simulink model "ABS_Regen_SLC_Test"  (R2023a)
settings: Solver=ode45  StartTime=0  StopTime=15  FixedStep=0.002  RelTol=1e-3  AbsTol=1e-6
libraries: Solver_SF x1, cstblocks x1
settings Model: ExtModeTrigMode=oneshot  VariantFading=off  Creator=ywata  LastModifiedBy=cheho
settings SolverCC: AutoScaleAbsTol=off  AlgebraicLoopSolver=TrustRegion
settings DataIOCC: SaveFormat=Array  SignalLoggingSaveFormat=ModelDataLogs  ReturnWorkspaceOutputs=off  SignalLoggingName=sigsOut
settings OptimizationCC: BlockReduction=off  BooleanDataType=off  ExpressionDepthLimit=2147483647  LifeSpan=inf
settings DebuggingCC: SaveWithParameterizedLinksMsg=none  UnderspecifiedInitializationDetection=Classic  MergeDetectMultiDrivingBlocksExec=none  SignalResolutionControl=TryResolveAllWithWarning  MultiTaskDSMMsg=warning  MultiTaskCondExecSysMsg=none  FcnCallInpInsideContextMsg=warning  UnconnectedInputMsg=warning  UnconnectedOutputMsg=warning  UnconnectedLineMsg=warning  StateNameClashWarn=warning  SFUnexpectedBacktrackingDiag=warning  SFNoUnconditionalDefaultTransitionDiag=warning  SFExecutionAtInitializationDiag=none  ArithmeticOperatorsInVariantConditions=warning
settings HardwareCC: ProdBitPerPointer=32  ProdBitPerSizeT=32  ProdBitPerPtrDiffT=32  ProdLargestAtomicFloat=None  ProdIntDivRoundTo=Undefined  ProdEndianess=Unspecified  ProdWordSize=32  ProdHWDeviceType=32-bit Generic  TargetUnknown=on
settings ModelReferenceCC: PropagateSignalLabelsOutOfModel=off
settings SFSimCC: SimUseLocalCustomCode=off  CustomCodeUndefinedFunction=UseInterfaceOnly
settings RTWCC: TemplateMakefile=grt_vc.tmf  RTWUseLocalCustomCode=off
settings CodeAppCC: StateflowObjectComments=on
settings GRTTargetCC: TargetFcnLib=ansi_tfl_tmw.mat  TargetLangStandard=C89/C90 (ANSI)  CombineOutputUpdateFcns=off  GRTInterface=on
settings ConfigComp: CovMetricSettings=dw  CovSaveCumulativeToWorkspaceVar=on  CovSaveSingleToWorkspaceVar=on  CovExternalEMLEnable=off

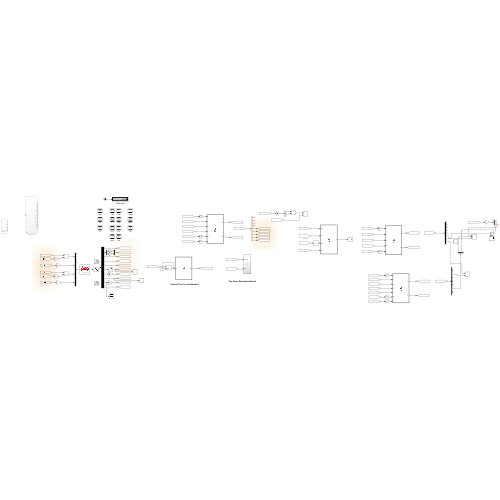
[thumbnail: Simulink's stored preview of the top-level diagram]
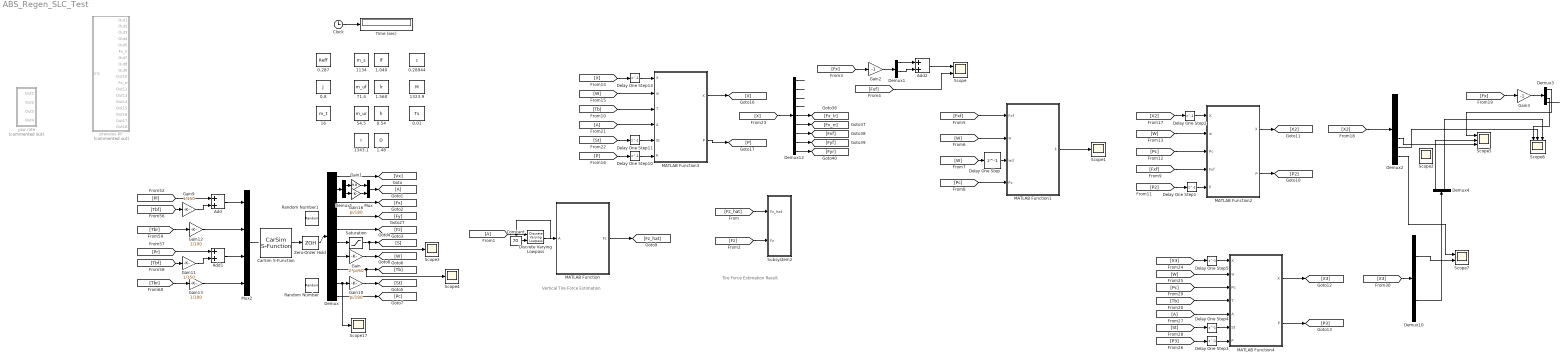
== system ABS_Regen_SLC_Test ==
  note: Vertical Tire Force Estimation
  note: Tire Force Estimation Result
  0.01 : DataStoreMemory  DataStoreName=Ts  WriteAfterWriteMsg=warning  InitialValue=0.01  ShowAdditionalParam=off  OutDataTypeStr=double
  0.287 : DataStoreMemory  DataStoreName=Reff  WriteAfterWriteMsg=warning  InitialValue=0.287  ShowAdditionalParam=off  OutDataTypeStr=double
  0.28944 : DataStoreMemory  DataStoreName=c  WriteAfterWriteMsg=warning  InitialValue=0.29844  ShowAdditionalParam=off  OutDataTypeStr=double
  0.54 : DataStoreMemory  DataStoreName=h  WriteAfterWriteMsg=warning  InitialValue=0.54  ShowAdditionalParam=off  OutDataTypeStr=double
  0.8 : DataStoreMemory  DataStoreName=J  WriteAfterWriteMsg=warning  InitialValue=0.8  ShowAdditionalParam=off  OutDataTypeStr=double
  1.040 : DataStoreMemory  DataStoreName=lf  WriteAfterWriteMsg=warning  InitialValue=1.040  ShowAdditionalParam=off  OutDataTypeStr=double
  1.48 : DataStoreMemory  DataStoreName=D  WriteAfterWriteMsg=warning  InitialValue=1.48  ShowAdditionalParam=off  OutDataTypeStr=double
  1.560 : DataStoreMemory  DataStoreName=lr  WriteAfterWriteMsg=warning  InitialValue=1.560  ShowAdditionalParam=off  OutDataTypeStr=double
  1134 : DataStoreMemory  DataStoreName=m_s  WriteAfterWriteMsg=warning  InitialValue=1134  ShowAdditionalParam=off  OutDataTypeStr=double
  1323.9 : DataStoreMemory  DataStoreName=M  WriteAfterWriteMsg=warning  InitialValue=1323.9  ShowAdditionalParam=off  OutDataTypeStr=double
  1343.1 : DataStoreMemory  DataStoreName=I  WriteAfterWriteMsg=warning  InitialValue=1343.1  ShowAdditionalParam=off  OutDataTypeStr=double
  16 : DataStoreMemory  DataStoreName=m_t  WriteAfterWriteMsg=warning  InitialValue=16  ShowAdditionalParam=off  OutDataTypeStr=double
  54.5 : DataStoreMemory  DataStoreName=m_ur  WriteAfterWriteMsg=warning  InitialValue=54.5  ShowAdditionalParam=off  OutDataTypeStr=double
  71.4 : DataStoreMemory  DataStoreName=m_uf  WriteAfterWriteMsg=warning  InitialValue=71.4  ShowAdditionalParam=off  OutDataTypeStr=double
  Add : Sum
  Add1 : Sum
  Add2 : Sum
  CarSim S-Function : Solver_SF/CarSim S-Function  Priority=1  SIMFILE=simfile.sim  Run_RTs=off  vs_state_ind=Run  StopMode_ind=Vehicle Model
  Clock : Clock
  Constant : Constant  Value=70  SampleTime=0.01
  Delay One Step : Delay  DelayLength=1  InitialCondition=[67.665 67.665 67.665 67.665]'
  Delay One Step1 : Delay  DelayLength=1  InitialCondition=diag([67.655 67.655 0 0 0 0 0])
  Delay One Step10 : Delay  DelayLength=1  InitialCondition=diag([67.655 67.655 0 0 0 0 0 0 0])
  Delay One Step11 : Delay  DelayLength=1  InitialCondition=[0 0]'
  Delay One Step14 : Delay  DelayLength=1  InitialCondition=[67.655 67.655 0 0 0 0 0 0 0]'
  Delay One Step2 : Delay  DelayLength=1  InitialCondition=[67.655 67.655 0 0 0 0 0]'
  Delay One Step3 : Delay  DelayLength=1  InitialCondition=diag([67.655 67.655 67.655 67.655 250 0 0 0 0 0 0 0 0 0 0 0])
  Delay One Step4 : Delay  DelayLength=1  InitialCondition=[0 0]'
  Delay One Step5 : Delay  DelayLength=1  InitialCondition=[67.655 67.655 67.655 67.655 100 0 0 0 0 0 0 0 0 0 0 0]'
  Demux : Demux  Outputs=[1 3 4 4 4 4 4 4 2 2]
  Demux1 : Demux
  Demux10 : Demux  Outputs=[4 1 2 1 2 4 2]
  Demux12 : Demux  Outputs=9
  Demux2 : Demux  Outputs=7
  Demux3 : Demux
  Demux4 : Demux
  Demux5 : Demux  Outputs=[2 1]
  Discrete Varying Lowpass : cstblocks/Linear Parameter Varying/Discrete Varying Lowpass  N=1  w0=0  Ts=0.01
  From1 : From
  From21 : From
  From27 : From
  Gain : Gain  Gain=2*pi/60
  Gain1 : Gain  Gain=9.8
  Gain10 : Gain  Gain=pi/180
  Gain11 : Gain  Gain=1/150
  Gain12 : Gain  Gain=1/100
  Gain13 : Gain  Gain=1/100
  Gain16 : Gain  Gain=pi/180
  Gain2 : Gain  Gain=-1
  Gain3 : Gain  Gain=-1
  Gain9 : Gain  Gain=1/150
  Goto1 : Goto
  MATLAB Function : MATLAB Function  TreatAsAtomicUnit=on
  MATLAB Function1 : MATLAB Function  TreatAsAtomicUnit=on
  MATLAB Function2 : MATLAB Function  TreatAsAtomicUnit=on
  MATLAB Function3 : MATLAB Function  TreatAsAtomicUnit=on
  MATLAB Function4 : MATLAB Function  TreatAsAtomicUnit=on
  Mux : Mux  Inputs=2
  Mux2 : Mux
  Random Number : RandomNumber  Variance=0.01^2  SampleTime=0.01
  Random Number1 : RandomNumber  Variance=0.01  SampleTime=0.01
  Saturation : Saturate  UpperLimit=1  LowerLimit=-1
  Scope : Scope  NumInputPorts=2
  Scope{1..4,17} (5 alike) : Scope
  Scope5 : Scope  NumInputPorts=3
  Scope6 : Scope  NumInputPorts=3
  Scope7 : Scope  NumInputPorts=2
  Subsystem2 : Subsystem
  Time (sec) : Display
      settings: Format=bank  Decimation=100
  Zero-Order Hold : ZeroOrderHold  SampleTime=0.01
  previous KF : Subsystem  Commented=on
  yaw rate : Subsystem  Commented=on
  wires:
  CarSim S-Function/1 -> Zero-Order Hold/1
  Clock/1 -> Time (sec)/1
  Demux/1 -> [Vx]
  Demux/3 -> [Fx]
  Zero-Order Hold/1 -> Demux/1
  Saturation/1 -> Scope3/1, [S]
  Gain/1 -> [W]
  Demux/2 -> Demux5/1
  Demux5/1 -> Gain1/1
  Mux/1 -> Goto1/1
  Demux5/2 -> Gain16/1
  Gain1/1 -> Mux/1
  Demux/10 -> [Pc]
  Demux/9 -> Scope17/1, Gain10/1
  Demux/8 -> Scope4/1, [Tb]
  Demux/7 -> Gain/1
  Demux/6 -> Saturation/1
  Demux/5 -> [Fz]
  Demux/4 -> [Fy]
  Gain16/1 -> Mux/2
  Gain10/1 -> [St]
  From1/1 -> MATLAB Function/1(A), Discrete Varying Lowpass/1
  MATLAB Function/1(Fz) -> [Fz_hat]
  [Fz_hat] -> Subsystem2/1(Fz_hat)
  [Fz] -> Subsystem2/2(Fz)
  Constant/1 -> Discrete Varying Lowpass/2
  Discrete Varying Lowpass/1 -> ?
  Add/1 -> Mux2/1
  [Pl] -> Add/1
  [Tbf] -> Gain9/1
  Gain9/1 -> Add/2
  [Tbf] -> Gain11/1
  Add1/1 -> Mux2/3
  [Pr] -> Add1/1
  Gain11/1 -> Add1/2
  [Tbr] -> Gain12/1
  Gain12/1 -> Mux2/2
  Gain13/1 -> Mux2/4
  [Tbr] -> Gain13/1
  Mux2/1 -> ?
  [P] -> Delay One Step10/1
  Demux12/3 -> ?
  [X] -> Demux12/1
  Demux12/1 -> ?
  Demux12/2 -> ?
  Delay One Step14/1 -> MATLAB Function3/1("X ")
  Demux12/4 -> ?
  Demux12/8 -> [Fyf]
  Demux12/9 -> [Fyr]
  Delay One Step10/1 -> MATLAB Function3/6("P ")
  Demux12/6 -> [Fx_rr]
  [Tb] -> MATLAB Function3/3(T)
  MATLAB Function3/2(P) -> [P]
  Delay One Step11/1 -> MATLAB Function3/5(St)
  [W] -> MATLAB Function3/2(w)
  MATLAB Function3/1(X) -> [X]
  [X] -> Delay One Step14/1
  Demux12/5 -> [Fx_lr]
  From21/1 -> MATLAB Function3/4(A)
  Demux12/7 -> [Fxf]
  [St] -> Delay One Step11/1
  [Fx] -> Gain2/1
  Demux1/1 -> Add2/1
  Demux1/3 -> Add2/2
  Add2/1 -> Scope/1
  Gain2/1 -> Demux1/1
  [Fxf] -> Scope/2
  [Fxf] -> MATLAB Function1/1(Fxf)
  [W] -> MATLAB Function1/2(w)
  [W] -> Delay One Step/1
  Delay One Step/1 -> MATLAB Function1/3(wd)
  [Pc] -> MATLAB Function1/4(Pc)
  MATLAB Function1/1(k) -> Scope1/1
  [Fxf] -> MATLAB Function2/4(Fxf)
  [P2] -> Delay One Step1/1
  Delay One Step1/1 -> MATLAB Function2/5("P ")
  MATLAB Function2/2(P) -> [P2]
  [Pc] -> MATLAB Function2/3(Pc)
  [W] -> MATLAB Function2/2(w)
  MATLAB Function2/1(X) -> [X2]
  [X2] -> Delay One Step2/1
  Delay One Step2/1 -> MATLAB Function2/1("X ")
  [X2] -> Demux2/1
  Demux2/7 -> Scope7/1
  Demux2/5 -> Scope5/3
  Gain3/1 -> Demux3/1
  [Fx] -> Gain3/1
  Demux2/6 -> Scope6/2
  Demux3/4 -> ?
  Demux3/3 -> Scope6/1
  Demux3/1 -> Scope5/1
  [P3] -> Delay One Step3/1
  [Tb] -> MATLAB Function4/4(T)
  [X3] -> Delay One Step5/1
  MATLAB Function4/2(P) -> [P3]
  Delay One Step5/1 -> MATLAB Function4/1("X ")
  MATLAB Function4/1(X) -> [X3]
  From27/1 -> MATLAB Function4/5(A)
  [St] -> Delay One Step4/1
  [Pc] -> MATLAB Function4/3(Pc)
  Delay One Step4/1 -> MATLAB Function4/6(St)
  [W] -> MATLAB Function4/2(w)
  Delay One Step3/1 -> MATLAB Function4/7("P ")
  [X3] -> Demux10/1
  Demux10/2 -> Scope7/2
  Demux10/6 -> Demux4/1
  Demux4/1 -> Scope5/2
  Demux4/3 -> Scope6/3

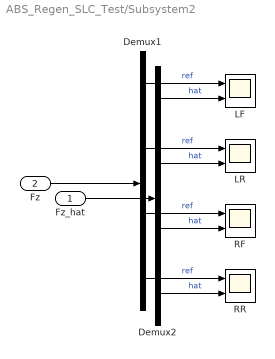
== system ABS_Regen_SLC_Test/Subsystem2 ==
  Fz_hat : Inport
  Fz : Inport  Port=2
  Demux1 : Demux
  Demux2 : Demux
  LF : Scope  NumInputPorts=2
  LR : Scope  NumInputPorts=2
  RF : Scope  NumInputPorts=2
  RR : Scope  NumInputPorts=2
  wires:
  Fz_hat/1 -> Demux2/1
  Fz/1 -> Demux1/1
  Demux1/1 -> LF/1  "ref"
  Demux2/1 -> LF/2  "hat"
  Demux2/2 -> LR/2  "hat"
  Demux1/2 -> LR/1  "ref"
  Demux1/3 -> RF/1  "ref"
  Demux2/3 -> RF/2  "hat"
  Demux1/4 -> RR/1  "ref"
  Demux2/4 -> RR/2  "hat"

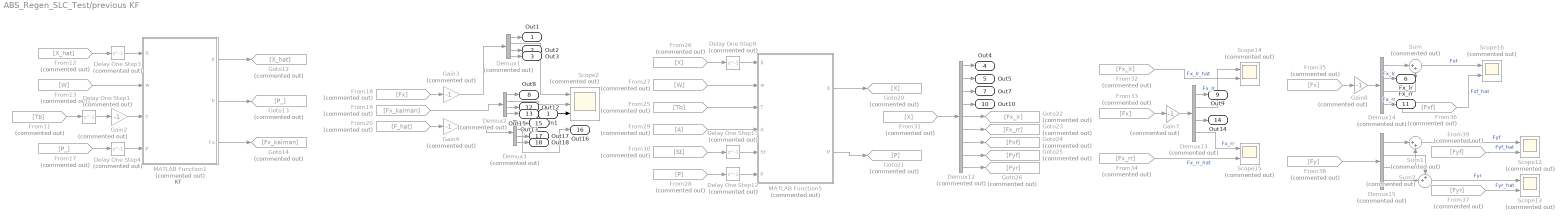
== system ABS_Regen_SLC_Test/previous KF ==
  note: KF
  In1 : Inport
  Delay One Step1 : Delay  Commented=on  DelayLength=1  InitialCondition=zeros(4,1)
  Delay One Step12 : Delay  Commented=on  DelayLength=1  InitialCondition=diag([67.655 67.655 0 0 0 0 0 0 0])
  Delay One Step13 : Delay  Commented=on  DelayLength=1  InitialCondition=[0 0]'
  Delay One Step3 : Delay  Commented=on  DelayLength=1  InitialCondition=[67.655 67.655 67.655 67.655; 0 0 0 0]
  Delay One Step4 : Delay  Commented=on  DelayLength=1  InitialCondition=10*ones(2,8)
  Delay One Step9 : Delay  Commented=on  DelayLength=1  InitialCondition=[67.655 67.655 0 0 0 0 0 0 0]'
  Demux{1..3,13..15} (6 alike) : Demux  Commented=on
  Demux12 : Demux  Commented=on  Outputs=9
  From11 : From  Commented=on  GotoTag=Tb
  From12 : From  Commented=on  GotoTag=X_hat
  From13 : From  Commented=on  GotoTag=W
  From17 : From  Commented=on  GotoTag=P_
  From18 : From  Commented=on  GotoTag=Fx
  From19 : From  Commented=on  GotoTag=Fx_kalman
  From20 : From  Commented=on  GotoTag=F_hat
  From25 : From  Commented=on  GotoTag=Tb
  From26 : From  Commented=on  GotoTag=X
  From27 : From  Commented=on  GotoTag=W
  From28 : From  Commented=on  GotoTag=P
  From29 : From  Commented=on
  From30 : From  Commented=on  GotoTag=St
  From31 : From  Commented=on  GotoTag=X
  From32 : From  Commented=on  GotoTag=Fx_lr
  From33 : From  Commented=on  GotoTag=Fx
  From34 : From  Commented=on  GotoTag=Fx_rr
  From35 : From  Commented=on  GotoTag=Fx
  From36 : From  Commented=on  GotoTag=Fxf
  From37 : From  Commented=on  GotoTag=Fyr
  From38 : From  Commented=on  GotoTag=Fy
  From39 : From  Commented=on  GotoTag=Fyf
  Gain{2..4,7..8} (5 alike) : Gain  Commented=on  Gain=-1
  Goto12 : Goto  Commented=on  GotoTag=X_hat
  Goto13 : Goto  Commented=on  GotoTag=P_
  Goto14 : Goto  Commented=on  GotoTag=Fx_kalman
  Goto20 : Goto  Commented=on  GotoTag=X
  Goto21 : Goto  Commented=on  GotoTag=P
  Goto22 : Goto  Commented=on  GotoTag=Fx_lr
  Goto23 : Goto  Commented=on  GotoTag=Fx_rr
  Goto24 : Goto  Commented=on  GotoTag=Fxf
  Goto25 : Goto  Commented=on  GotoTag=Fyf
  Goto26 : Goto  Commented=on  GotoTag=Fyr
  MATLAB Function1 : MATLAB Function  Commented=on  TreatAsAtomicUnit=on
  MATLAB Function5 : MATLAB Function  Commented=on  TreatAsAtomicUnit=on
  Scope{12..16} (5 alike) : Scope  Commented=on  NumInputPorts=2
  Scope2 : Scope  Commented=on  NumInputPorts=3
  Sum : Sum  Commented=on  Inputs=|++
  Sum1 : Sum  Commented=on  Inputs=|++
  Sum2 : Sum  Commented=on  Inputs=++|
  Out1 : Outport
  Out2 : Outport  Port=2
  Out3 : Outport  Port=3
  Out4 : Outport  Port=4
  Out5 : Outport  Port=5
  Fx_lr : Outport  Port=6
  Out7 : Outport  Port=7
  Out8 : Outport  Port=8
  Out9 : Outport  Port=9
  Out10 : Outport  Port=10
  Fx_rr : Outport  Port=11
  Out12 : Outport  Port=12
  Out13 : Outport  Port=13
  Out14 : Outport  Port=14
  Out15 : Outport  Port=15
  Out16 : Outport  Port=16
  Out17 : Outport  Port=17
  Out18 : Outport  Port=18
  wires:
  From26/1 -> Delay One Step9/1
  Demux12/7 -> Goto24/1
  Delay One Step4/1 -> MATLAB Function1/4("P ")
  MATLAB Function5/1(X) -> Goto20/1
  Demux2/1 -> Out8/1
  Demux3/1 -> Out15/1
  Demux1/2 -> Scope2/1
  MATLAB Function1/2(P) -> Goto13/1
  From27/1 -> MATLAB Function5/2(w)
  Gain3/1 -> Demux1/1
  Delay One Step3/1 -> MATLAB Function1/1("X ")
  Sum1/1 -> Scope12/1  "Fyf"
  MATLAB Function1/1(X) -> Goto12/1
  From13/1 -> MATLAB Function1/2(w)
  From20/1 -> Gain4/1
  Demux2/3 -> Out12/1
  Demux2/2 -> Scope2/2
  From29/1 -> MATLAB Function5/4(A)
  Delay One Step1/1 -> Gain2/1
  From11/1 -> Delay One Step1/1
  Demux15/3 -> Sum1/2
  Demux13/3 -> Out14/1
  From12/1 -> Delay One Step3/1
  From35/1 -> Gain8/1
  Gain4/1 -> Demux3/1
  Demux13/1 -> Out9/1
  Demux13/2 -> Scope14/1  "Fx_lr"
  From30/1 -> Delay One Step13/1
  From38/1 -> Demux15/1
  Demux12/4 -> Out10/1
  From33/1 -> Gain7/1
  Gain7/1 -> Demux13/1
  From31/1 -> Demux12/1
  Sum/1 -> Scope16/1  "Fxf"
  Delay One Step12/1 -> MATLAB Function5/6("P ")
  Demux13/4 -> Scope15/1  "Fx_rr"
  Demux14/3 -> Sum/2
  MATLAB Function5/2(P) -> Goto21/1
  From32/1 -> Scope14/2  "Fx_lr_hat"
  Demux2/4 -> Out13/1
  From19/1 -> Demux2/1
  From17/1 -> Delay One Step4/1
  Demux12/5 -> Goto22/1
  From37/1 -> Scope13/2  "Fyr_hat"
  Demux14/1 -> Sum/1
  From36/1 -> Scope16/2  "Fxf_hat"
  Demux15/4 -> Sum2/2
  From25/1 -> MATLAB Function5/3(T)
  Demux12/8 -> Goto25/1
  Gain8/1 -> Demux14/1
  MATLAB Function1/3(Fx) -> Goto14/1
  Sum2/1 -> Scope13/1  "Fyr"
  From34/1 -> Scope15/2  "Fx_rr_hat"
  From18/1 -> Gain3/1
  Demux12/1 -> Out4/1
  Demux15/1 -> Sum1/1
  From28/1 -> Delay One Step12/1
  Delay One Step13/1 -> MATLAB Function5/5(St)
  Demux3/3 -> Out17/1
  From39/1 -> Scope12/2  "Fyf_hat"
  Demux3/2 -> Out16/1
  Demux12/9 -> Goto26/1
  Demux15/2 -> Sum2/1
  Delay One Step9/1 -> MATLAB Function5/1("X ")
  Demux12/6 -> Goto23/1
  Demux14/2 -> Fx_lr/1  "Fx_lr"
  Gain2/1 -> MATLAB Function1/3(T)
  Demux14/4 -> Fx_rr/1  "Fx_rr"
  Demux3/4 -> Out18/1
  Demux1/1 -> Out1/1
  Demux1/3 -> Out2/1
  Demux1/4 -> Out3/1
  Demux12/2 -> Out5/1
  In1/1 -> Scope2/3
  Demux12/3 -> Out7/1

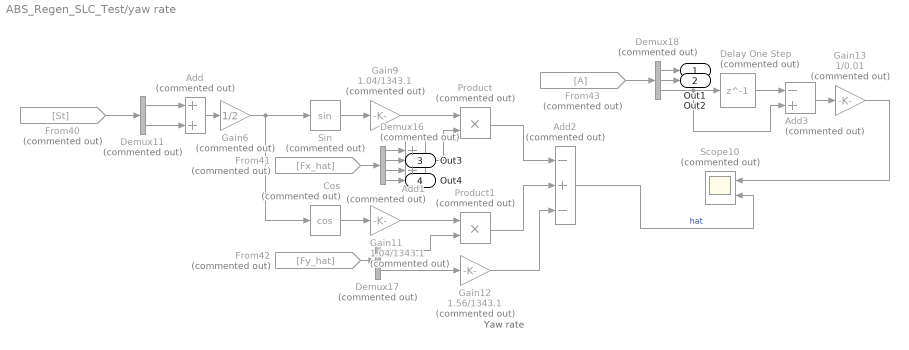
== system ABS_Regen_SLC_Test/yaw rate ==
  note: Yaw rate
  Add : Sum  Commented=on
  Add1 : Sum  Commented=on
  Add2 : Sum  Commented=on  Inputs=-+-
  Add3 : Sum  Commented=on  Inputs=-+
  Cos : Trigonometry  Commented=on  Operator=cos
  Delay One Step : Delay  Commented=on  DelayLength=1
  Demux11 : Demux  Commented=on  Outputs=2
  Demux16 : Demux  Commented=on
  Demux17 : Demux  Commented=on  Outputs=2
  Demux18 : Demux  Commented=on  Outputs=3
  From40 : From  Commented=on  GotoTag=St
  From41 : From  Commented=on  GotoTag=Fx_hat
  From42 : From  Commented=on  GotoTag=Fy_hat
  From43 : From  Commented=on
  Gain11 : Gain  Commented=on  Gain=1.04/1343.1
  Gain12 : Gain  Commented=on  Gain=1.56/1343.1
  Gain13 : Gain  Commented=on  Gain=1/0.01
  Gain6 : Gain  Commented=on  Gain=1/2
  Gain9 : Gain  Commented=on  Gain=1.04/1343.1
  Product : Product  Commented=on
  Product1 : Product  Commented=on
  Scope10 : Scope  Commented=on  NumInputPorts=2
  Sin : Trigonometry  Commented=on
  Out1 : Outport
  Out2 : Outport  Port=2
  Out3 : Outport  Port=3
  Out4 : Outport  Port=4
  wires:
  Gain6/1 -> Cos/1, Sin/1
  Cos/1 -> Gain11/1
  Add1/1 -> Product/2
  Product1/1 -> Add2/2
  Gain9/1 -> Product/1
  Demux16/1 -> Add1/1
  Demux17/1 -> Product1/2
  Demux17/2 -> Gain12/1
  Gain12/1 -> Add2/3
  Add3/1 -> Gain13/1
  Demux18/3 -> Add3/2, Delay One Step/1
  Demux16/2 -> Out3/1
  Gain13/1 -> Scope10/1
  Add2/1 -> Scope10/2  "hat"
  Product/1 -> Add2/1
  Demux18/1 -> Out1/1
  Delay One Step/1 -> Add3/1
  Sin/1 -> Gain9/1
  Demux16/3 -> Add1/2
  From41/1 -> Demux16/1
  Gain11/1 -> Product1/1
  Demux11/1 -> Add/1
  From42/1 -> Demux17/1
  Demux18/2 -> Out2/1
  Demux11/2 -> Add/2
  Demux16/4 -> Out4/1
  Add/1 -> Gain6/1
  From43/1 -> Demux18/1
  From40/1 -> Demux11/1

== matlab function ABS_Regen_SLC_Test/previous KF/MATLAB Function5 ==
  data: X input; w input; T input; A input; St input; X output; P output; P input; Reff data_store_memory; J data_store_memory; Ts data_store_memory; I data_store_memory; M data_store_memory; lf data_store_memory; lr data_store_memory
function [X,P]  = fcn(X,w,T,A,St,P)

global  Reff J Ts I M lf lr;

delta = (St(1)+St(2))/2;

%X = [w_lr w_rr r T F_lr F_rr F_xf F_yf F_yr]
Q = diag([0.000001 0.0001 0.000001 1000 150 150 1000 50000 50000]);

%Z = [w_lr w_rr r T ax ay]
Z = [w(2),w(4),A(3),-T(2),A(1),A(2)]';
R = diag([0.00028 0.00028 0.0000001 0.1 0.001 0.001]);

F = eye(9) + Ts*...
    [0 0 0 -1/J Reff/J 0 0 0 0;
     0 0 0 -1/J 0 Reff/J 0 0 0;
     0 0 0 0 0 0 -lf*sin(delta)/I lf*cos(delta)/I -lr/I;
     zeros(6,9)];

H = [1 0 0 0 0 0 0 0 0;
     0 1 0 0 0 0 0 0 0;
     0 0 1 0 0 0 0 0 0;
     0 0 0 1 0 0 0 0 0;
     0 0 0 0 -1/M -1/M -cos(delta)/M -sin(delta)/M 0;
     0 0 0 0 0 0 -sin(delta)/M cos(delta)/M 1/M];

Xm = F*X;
Pm = F*P*F'+Q;
K = Pm*H'/(H*Pm*H'+R);
X = Xm+K*(Z-H*Xm);
P = (eye(9)-K*H)*Pm;

end

== matlab function ABS_Regen_SLC_Test/MATLAB Function2 ==
  data: X input; w input; Pc input; Fxf input; X output; P output; P input; Reff data_store_memory; J data_store_memory; Ts data_store_memory; I data_store_memory; M data_store_memory; lf data_store_memory; lr data_store_memory
function [X,P]  = fcn(X,w,Pc,Fxf,P)

global  Reff J Ts I M lf lr;

%X = [w_lf w_rf Pl Pr F_lr F_rr k]
Q = diag([0.000001 0.0001 0.01 0.01 150 150 1]);

%Z = [w_lf w_rf Pl Pr Fxf]
Z = [w(1),w(3),Pc(1),Pc(2),Fxf]';
R = diag([0.00028 0.00028 0.01 0.01 0.1]);

F = eye(7) + Ts*...
    [0 0 -1/J*X(7) 0 Reff/J 0 -1/J*X(3);
     0 0 0 -1/J*X(7) 0 Reff/J -1/J*X(4);
     zeros(5,7)];

H = [1 0 0 0 0 0 0;
     0 1 0 0 0 0 0;
     0 0 1 0 0 0 0;
     0 0 0 1 0 0 0;
     0 0 0 0 1 1 0;];

Xm = [X(1)+Ts/J*(Reff*X(5)-X(3)*X(7));
      X(2)+Ts/J*(Reff*X(6)-X(4)*X(7));
      X(3);X(4);X(5);X(6);X(7);];
Pm = F*P*F'+Q;
K = Pm*H'/(H*Pm*H'+R);
X = Xm+K*(Z-H*Xm);
P = (eye(7)-K*H)*Pm;

end

== matlab function ABS_Regen_SLC_Test/MATLAB Function4 ==
  data: X input; w input; Pc input; T input; A input; St input; X output; P output; P input; Reff data_store_memory; J data_store_memory; Ts data_store_memory; I data_store_memory; M data_store_memory; lf data_store_memory; lr data_store_memory
function [X,P]  = fcn(X,w,Pc,T,A,St,P)

global  Reff J Ts I M lf lr;
T(1) = 0;
delta = (St(1)+St(2))/2;

%X = [w_lf w_lr w_rf w_rr k Pl Pr r Tf Tr F_lf F_lr F_rf F_rr F_yf F_yr]
Q = diag([0.00001 0.00001 0.00001 0.00001 0.000001 1000 1000 0.000001 1000 1000 100 100 100 100 1000 1000]);

%Z = [w_lf w_lr w_rf w_rr Pl Pr r Tf Tr ax ay]
Z = [w(1),w(2),w(3),w(4),Pc(1),Pc(2),A(3),-T(1),-T(2),A(1),A(2)]';
R = diag([0.00028 0.00028 0.00028 0.00028 0.01 0.01 0.0000001 0.001 0.001 0.0001 0.0001]);

F = eye(16) + Ts*...
    [0 0 0 0 -1/J*X(6) -1/J*X(5) 0 0 -1/J 0 Reff/J 0 0 0 0 0;
     0 0 0 0 0 0 0 0 0 -1/J 0 Reff/J 0 0 0 0;
     0 0 0 0 -1/J*X(7) 0 -1/J*X(5) 0 -1/J 0 0 0 Reff/J 0 0 0;
     0 0 0 0 0 0 0 0 0 -1/J 0 0 0 Reff/J 0 0;
     zeros(3,16);
     0 0 0 0 0 0 0 0 0 0 -lf/I*sin(delta) 0 -lf/I*sin(delta) 0 lf/I*cos(delta) -lr/I;
     zeros(8,16)];

H = [1 0 0 0 0 0 0 0 0 0 0 0 0 0 0 0;
     0 1 0 0 0 0 0 0 0 0 0 0 0 0 0 0;
     0 0 1 0 0 0 0 0 0 0 0 0 0 0 0 0;
     0 0 0 1 0 0 0 0 0 0 0 0 0 0 0 0;
     0 0 0 0 0 1 0 0 0 0 0 0 0 0 0 0;
     0 0 0 0 0 0 1 0 0 0 0 0 0 0 0 0;
     0 0 0 0 0 0 0 1 0 0 0 0 0 0 0 0;
     0 0 0 0 0 0 0 0 1 0 0 0 0 0 0 0;
     0 0 0 0 0 0 0 0 0 1 0 0 0 0 0 0;
     0 0 0 0 0 0 0 0 0 0 -cos(delta)/M -1/M -cos(delta)/M -1/M -sin(delta)/M 0;
     0 0 0 0 0 0 0 0 0 0 -sin(delta)/M 0 -sin(delta)/M 0 cos(delta)/M 1/M];

X(1) = X(1) + (Reff/J*X(11)-1/J*(X(5)*X(6)+X(9)))*Ts;
X(2) = X(2) + (Reff/J*X(12)-1/J*X(10))*Ts;
X(3) = X(3) + (Reff/J*X(13)-1/J*(X(5)*X(7)+X(9)))*Ts;
X(4) = X(4) + (Reff/J*X(14)-1/J*X(10))*Ts;
X(8) = X(8) + (-lf/I*sin(delta)*(X(11)+X(13))+lf/I*cos(delta)*X(15)-lr/I*X(16))*Ts;



Xm = X;
Pm = F*P*F'+Q;
K = Pm*H'/(H*Pm*H'+R);
X = Xm+K*(Z-H*Xm);
P = (eye(16)-K*H)*Pm;

end

== matlab function ABS_Regen_SLC_Test/previous KF/MATLAB Function1 ==
  data: X input; w input; T input; X output; P output; P input; Fx output; Reff data_store_memory; J data_store_memory; Ts data_store_memory
function [X,P,Fx]  = fcn(X,w,T,P)

global  Reff J Ts;

Qlf = [1 0;0 500000]; Qlr = [0.01 0;0 900]; Qrf = [1 0;0 500000]; Qrr = [1 0;0 500000]; Q = [Qlf Qlr Qrf Qrr];
Rlf = 1; Rlr = 0.01; Rrf = 1; Rrr = 1; R = [Rlf Rlr Rrf Rrr];

F = [1 Reff/J*Ts;0 1]; G = [-1/J*Ts;0]; H = [1 0];

for i = 1:4
    xm = F*X(:,i)+G*T(i);
    Pm = F*P(:,2*i-1:2*i)*F'+Q(:,2*i-1:2*i);
    K = Pm*H'/(H*Pm*H'+R(i));
    X(:,i) = xm+K*(w(i)-H*xm);
    P(:,2*i-1:2*i) = (eye(2)-K*H)*Pm;
end
Fx = X(2,:);

== matlab function ABS_Regen_SLC_Test/MATLAB Function ==
  data: A input; Fz output; m_s data_store_memory; m_uf data_store_memory; m_ur data_store_memory; lf data_store_memory; lr data_store_memory; h data_store_memory; m_t data_store_memory; D data_store_memory
function Fz = fcn(A)

a = [9.8 A(1) A(2)]';

global m_s m_uf m_ur lf lr h m_t D

L = lf+lr;
Mz = [lr/(2*L)*m_s+1/2*m_uf+m_t -h/(2*L)*m_s -h/(2*D)*m_s;
     lf/(2*L)*m_s+1/2*m_ur+m_t h/(2*L)*m_s -h/(2*D)*m_s;
     lr/(2*L)*m_s+1/2*m_uf+m_t -h/(2*L)*m_s h/(2*D)*m_s;
     lf/(2*L)*m_s+1/2*m_ur+m_t h/(2*L)*m_s h/(2*D)*m_s];

Fz = Mz*a;

== matlab function ABS_Regen_SLC_Test/MATLAB Function3 ==
  data: X input; w input; T input; A input; St input; X output; P output; P input; Reff data_store_memory; J data_store_memory; Ts data_store_memory; I data_store_memory; M data_store_memory; lf data_store_memory; lr data_store_memory
function [X,P]  = fcn(X,w,T,A,St,P)

global  Reff J Ts I M lf lr;

delta = (St(1)+St(2))/2;

%X = [w_lr w_rr r T F_lr F_rr F_xf F_yf F_yr]
Q = diag([0.000001 0.0001 0.000001 1000 150 150 1000 50000 50000]);

%Z = [w_lr w_rr r T ax ay]
Z = [w(2),w(4),A(3),-T(2),A(1),A(2)]';
R = diag([0.00028 0.00028 0.0000001 0.1 0.001 0.001]);

F = eye(9) + Ts*...
    [0 0 0 -1/J Reff/J 0 0 0 0;
     0 0 0 -1/J 0 Reff/J 0 0 0;
     0 0 0 0 0 0 -lf*sin(delta)/I lf*cos(delta)/I -lr/I;
     zeros(6,9)];

H = [1 0 0 0 0 0 0 0 0;
     0 1 0 0 0 0 0 0 0;
     0 0 1 0 0 0 0 0 0;
     0 0 0 1 0 0 0 0 0;
     0 0 0 0 -1/M -1/M -cos(delta)/M -sin(delta)/M 0;
     0 0 0 0 0 0 -sin(delta)/M cos(delta)/M 1/M];

Xm = F*X;
Pm = F*P*F'+Q;
K = Pm*H'/(H*Pm*H'+R);
X = Xm+K*(Z-H*Xm);
P = (eye(9)-K*H)*Pm;

end

== matlab function ABS_Regen_SLC_Test/MATLAB Function1 ==
  data: Fxf input; w input; wd input; Pc input; k output; Reff data_store_memory; J data_store_memory; Ts data_store_memory; I data_store_memory; M data_store_memory; lf data_store_memory; lr data_store_memory
function k   = fcn(Fxf,w,wd,Pc)

global  Reff J Ts I M lf lr;
wdot = w-wd;

k = (Fxf*Reff - J*(wdot(1)+wdot(3))/Ts)/(Pc(1)+Pc(2));

end
